simulink model "G_PC"  (R2019a)
settings: Solver=VariableStepAuto  StartTime=0.0  StopTime=10.0  RelTol=1e-3
undefined symbols (not defined in the file): GPC_B, Q_gP, T_gP, V_gPC, V_gPF
settings Model: Creator=rache  LastModifiedBy=rache
settings DataIOCC: ReturnWorkspaceOutputs=off
settings DebuggingCC: ArithmeticOperatorsInVariantConditions=warning

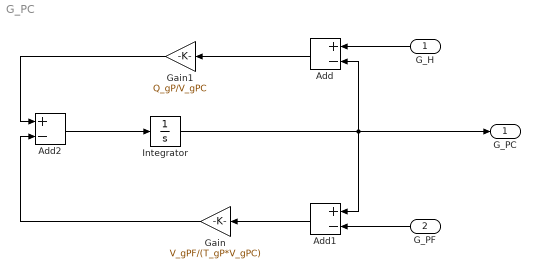
== system G_PC ==
  G_H : Inport
  G_PF : Inport  Port=2
  Add : Sum  Inputs=+-
  Add1 : Sum  Inputs=+-
  Add2 : Sum  Inputs=+-
  Gain : Gain  Gain=V_gPF/(T_gP*V_gPC)
  Gain1 : Gain  Gain=Q_gP/V_gPC
  Integrator : Integrator  InitialCondition=GPC_B  LimitOutput=on  LowerSaturationLimit=0
  G_PC : Outport
  wires:
  Integrator/1 -> Add/2, Add1/1, G_PC/1
  G_H/1 -> Add/1
  G_PF/1 -> Add1/2
  Add/1 -> Gain1/1
  Add1/1 -> Gain/1
  Add2/1 -> Integrator/1
  Gain1/1 -> Add2/1
  Gain/1 -> Add2/2
